simulink model "C_robust_fullobserver_Integral_Tracker_controller_secondpoles_s"  (R2021b)
settings: Solver=VariableStepAuto  StartTime=0.0  StopTime=40  RelTol=1e-3
undefined symbols (not defined in the file): A, B, C, C_r, KI2_1, KI2_2, L2
settings Model: Creator=nima8  LastModifiedBy=nima8

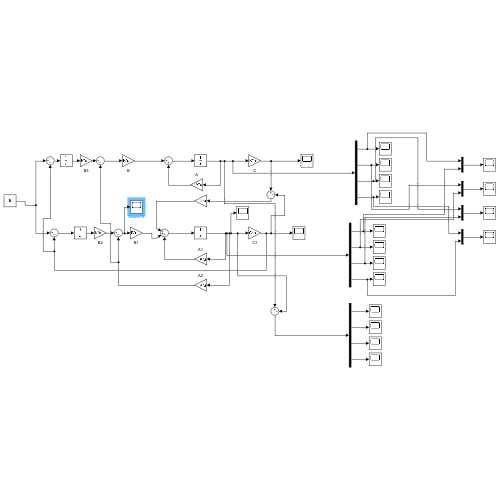
[thumbnail: Simulink's stored preview of the top-level diagram]
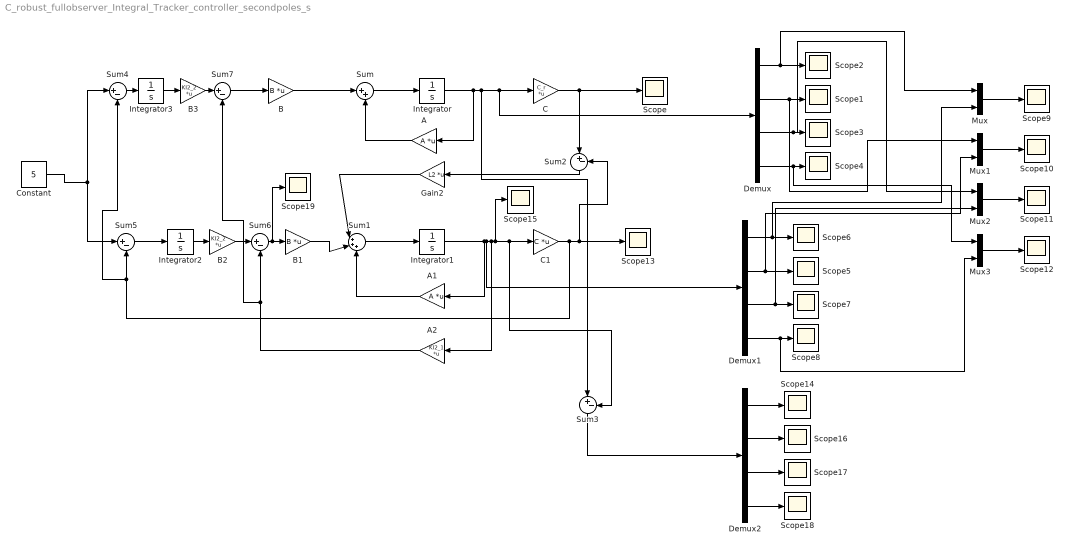
== system C_robust_fullobserver_Integral_Tracker_controller_secondpoles_s ==
  A : Gain  Gain=A  Multiplication=Matrix(K*u)
  A1 : Gain  Gain=A  Multiplication=Matrix(K*u)
  A2 : Gain  Gain=KI2_1  Multiplication=Matrix(K*u)
  B : Gain  Gain=B  Multiplication=Matrix(K*u)
  B1 : Gain  Gain=B  Multiplication=Matrix(K*u)
  B2 : Gain  Gain=KI2_2  Multiplication=Matrix(K*u)
  B3 : Gain  Gain=KI2_2  Multiplication=Matrix(K*u)
  C : Gain  Gain=C_r  Multiplication=Matrix(K*u)
  C1 : Gain  Gain=C  Multiplication=Matrix(K*u)
  Constant : Constant  Value=5
  Demux : Demux
  Demux1 : Demux
  Demux2 : Demux
  Gain2 : Gain  Gain=L2  Multiplication=Matrix(K*u)
  Integrator : Integrator  InitialCondition=[1 0.5 -1 2]
  Integrator1 : Integrator  InitialCondition=[-3 -2 3 -2]
  Integrator2 : Integrator  InitialCondition=1
  Integrator3 : Integrator  InitialCondition=1
  Mux{,1..3} (4 alike) : Mux  Inputs=2
  Scope{,1..19} (20 alike) : Scope
  Sum : Sum  Inputs=|++
  Sum1 : Sum  Inputs=|+++
  Sum{2..7} (6 alike) : Sum  Inputs=|+-
  wires:
  Integrator/1 -> Sum3/1, Demux/1, C/1, A/1
  Mux/1 -> Scope9/1
  Constant/1 -> Sum5/1, Sum4/1
  Demux2/2 -> Scope16/1
  Sum2/1 -> Gain2/1
  Mux3/1 -> Scope12/1
  Mux1/1 -> Scope10/1
  A/1 -> Sum/2
  Demux1/2 -> Mux1/2, Scope5/1
  Demux1/4 -> Mux3/2, Scope8/1
  Mux2/1 -> Scope11/1
  A1/1 -> Sum1/3
  Sum3/1 -> Demux2/1
  Demux/1 -> Mux/1, Scope2/1
  Demux/4 -> Mux3/1, Scope4/1
  Demux1/3 -> Mux2/2, Scope7/1
  Demux/2 -> Mux1/1, Scope1/1
  Demux2/4 -> Scope18/1
  C/1 -> Sum2/1, Scope/1
  Sum/1 -> Integrator/1
  Sum1/1 -> Integrator1/1
  B1/1 -> Sum1/2
  Demux1/1 -> Mux/2, Scope6/1
  B/1 -> Sum/1
  Demux2/1 -> Scope14/1
  Integrator1/1 -> A1/1, Demux1/1, A2/1, Scope15/1, Sum3/2, C1/1
  C1/1 -> Sum4/2, Sum5/2, Scope13/1, Sum2/2
  Demux2/3 -> Scope17/1
  Gain2/1 -> Sum1/1
  Demux/3 -> Mux2/1, Scope3/1
  Integrator2/1 -> B2/1
  B2/1 -> Sum6/1
  A2/1 -> Sum7/2, Sum6/2
  Sum7/1 -> B/1
  Sum4/1 -> Integrator3/1
  Integrator3/1 -> B3/1
  B3/1 -> Sum7/1
  Sum5/1 -> Integrator2/1
  Sum6/1 -> Scope19/1, B1/1
